simulink model "Temperature"  (R2020a)
settings: Solver=VariableStepAuto  StartTime=0.0  StopTime=10.0  RelTol=1e-3
libraries: arduinolib x1, simulink_extras x1
settings Model: Creator=pc  LastModifiedBy=pc

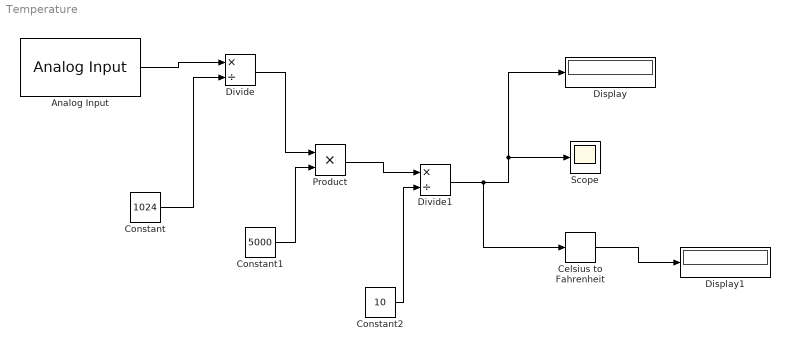
== system Temperature ==
  Analog Input : arduinolib/Analog Input  pinNumber=4  ReadResultsOnly=off  ConversionTriggerSource=Software  ExternalTriggerType=uint32( 0 )  OutputDataType=uint16  EnableConversionCompleteNotify=off  EnableOuputStatus=off  SampleTime=-1  blockPlatform=arduino
  Celsius to Fahrenheit : simulink_extras/Transformations/Celsius to Fahrenheit
      settings: SourceProductBaseCode=SL
  Constant : Constant  Value=1024
  Constant1 : Constant  Value=5000
  Constant2 : Constant  Value=10
  Display : Display
  Display1 : Display
  Divide : Product  Inputs=*/
  Divide1 : Product  Inputs=*/
  Product : Product
  Scope : Scope
  wires:
  Analog Input/1 -> Divide/1
  Constant/1 -> Divide/2
  Divide/1 -> Product/1
  Constant1/1 -> Product/2
  Constant2/1 -> Divide1/2
  Product/1 -> Divide1/1
  Divide1/1 -> Celsius to Fahrenheit/1, Scope/1, Display/1
  Celsius to Fahrenheit/1 -> Display1/1
